simulink model "Copy_of_control_main"  (R2026a)
settings: Solver=VariableStepAuto  StopTime=inf  FixedStep=0.01
values from neighbouring files (symbols this model uses):
  coefficients = [20.111978783 20.2762923351 20.4770477048]    [sensor_calibration.mat]
undefined symbols (not defined in the file or in its folder): az, Q
libraries: instrumentseriallib x3
settings Model: Creator=user  LastModifiedBy=user

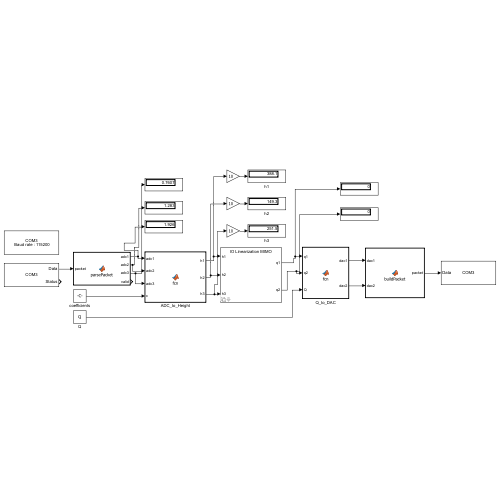
[thumbnail: Simulink's stored preview of the top-level diagram]
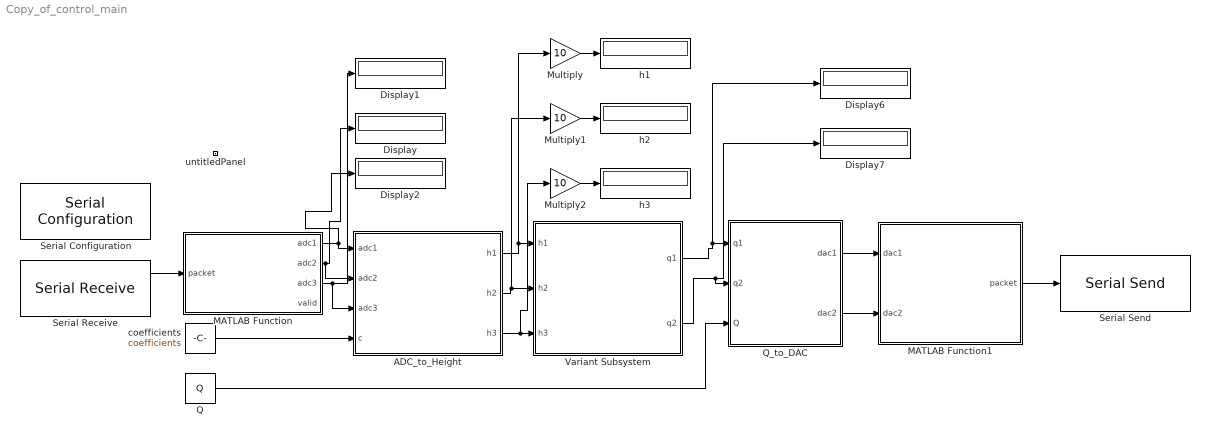
== system Copy_of_control_main ==
  ADC_to_Height : MATLAB Function  TreatAsAtomicUnit=on
  Display{,1..2,6..7} (5 alike) : Display
  MATLAB Function : MATLAB Function  TreatAsAtomicUnit=on
  MATLAB Function1 : MATLAB Function  TreatAsAtomicUnit=on
  Multiply : Gain  Gain=10
  Multiply1 : Gain  Gain=10
  Multiply2 : Gain  Gain=10
  Q : Constant  Value=Q
  Q_to_DAC : MATLAB Function  TreatAsAtomicUnit=on
  Serial Configuration : instrumentseriallib/Serial Configuration  Priority=-200000  PortSel=COM3  Port=COM3  ComPort=COM3  BaudRate=115200  DataBits=8  Parity=none  StopBits=1  ByteOrder=little-endian  FlowControl=none  Timeout=10  SimulateUsing=Interpreted execution  BlockInModel=on  aMode=1
  Serial Receive : instrumentseriallib/Serial Receive  Priority=1  PortSel=COM3  Port=COM3  ComPort=COM3  DataType=uint8  SaveDataType=uint8  ToggleHeader=on  Header=[0xAA 0x01]  ToggleDataSize=on  DataSize=[7]  ToggleTerminator=off  Terminator=<none>  CustomTerminator=[]  InputFormat=Column major  EnableBlockingMode=off  ActionDataUnavailable=Output last received value  ActionWhenDataUnavailable=Output last received value  CustomValue=0  SampleTime=0.01  SimulateUsing=Interpreted execution  BlockInModel=on  aMode=1  LibraryInUse=instrumentlib
  Serial Send : instrumentseriallib/Serial Send  Priority=1  PortSel=COM3  Port=COM3  ComPort=COM3  Header=[]  Terminator=<none>  CustomTerminator=[]  EnableBlockingMode=off  SimulateUsing=Interpreted execution  BlockInModel=on  aMode=1
  Variant Subsystem : Subsystem  Variant=on  mask{ctrl_mode=IO Linearization MIMO, r1=35, r2=25, r3=25, Kp_PI=10, Ki_PI=1, Kp1_PI=10, Ki1_PI=1, Kp2_PI=9, Ki2_PI=0.09, Kp_IO=0.5, Kp1_IO=1, Kp3_IO=15, Kp1_LIO=0, Kp3_LIO=0, Kd3_LIO=0, K_BS=1, Kz_BS=1, K1_BS=1, K3_BS=1, Kz_LBS=0, K1_LBS=0, K3_LBS=0, S1=10, S2=1, S3=10, R1_MPC=0.005, R2_MPC=0.005, H=40, S1_LMPC=10, S2_LMPC=1, S3_LMPC=10, R1_LMPC=0.005, R2_LMPC=0.005, H_LMPC=40}
      mask prompts: r1 "Tank1"; r2 "Tank2"; r3 "Tank3"; Kp_PI "Kp"; Ki_PI "Ki"; Kp1_PI "Kp1"; Ki1_PI "Ki1"; Kp2_PI "Kp2"; Ki2_PI "Ki2"; Kp_IO "Kp"; Kp1_IO "Kp1"; Kp3_IO "Kp3"; Kp1_LIO "Kp1"; Kp3_LIO "Kp3"; Kd3_LIO "Kd3"; K_BS "K"; Kz_BS "Kz"; K1_BS "K1"; K3_BS "K3"; Kz_LBS "Kz"; K1_LBS "K1"; K3_LBS "K3"; R1_MPC "R1"; R2_MPC "R2"; S1_LMPC "S1"; S2_LMPC "S2"; S3_LMPC "S3"; R1_LMPC "R1"; R2_LMPC "R2"; H_LMPC "H"
      mask DialogControl ParameterGroupVar Prompt: Controller
      mask DialogControl Container4 Prompt: Reference Levels
      mask DialogControl Container5 Prompt: PI SISO Parameters
      mask DialogControl Container6 Prompt: PI MIMO Parameters
      mask DialogControl Container7 Prompt: IO Linearization SISO
      mask DialogControl Container8 Prompt: IO Linearization MIMO
      mask DialogControl Container14 Prompt: Learning based IO Linearization MIMO
      mask DialogControl Container9 Prompt: Backstepping SISO
      mask DialogControl Container10 Prompt: Backstepping MIMO
      mask DialogControl Container13 Prompt: Learning based Backstepping MIMO
      mask DialogControl Container11 Prompt: MPC
      mask DialogControl Container12 Prompt: Learning based MPC
      mask DialogControl Container15 Prompt: RL
  coefficients : Constant  Value=coefficients
  h1 : Display
  h2 : Display
  h3 : Display
  untitledPanel : Subsystem  Tag=HiddenForWebPanel  IsWebBlockPanel=on
  wires:
  MATLAB Function1/1(packet) -> Serial Send/1
  Serial Receive/1 -> MATLAB Function/1(packet)
  MATLAB Function/2(adc2) -> ADC_to_Height/2(adc2), Display/1
  MATLAB Function/3(adc3) -> ADC_to_Height/3(adc3), Display1/1
  coefficients/1 -> ADC_to_Height/4(c)
  Q_to_DAC/1(dac1) -> MATLAB Function1/1(dac1)
  Q_to_DAC/2(dac2) -> MATLAB Function1/2(dac2)
  Q/1 -> Q_to_DAC/3(Q)
  ADC_to_Height/2(h2) -> Multiply1/1, Variant Subsystem/2(h2)
  ADC_to_Height/3(h3) -> Multiply2/1, Variant Subsystem/3(h3)
  Variant Subsystem/1(q1) -> Display6/1, Q_to_DAC/1(q1)
  Variant Subsystem/2(q2) -> Display7/1, Q_to_DAC/2(q2)
  MATLAB Function/1(adc1) -> ADC_to_Height/1(adc1), Display2/1
  Multiply/1 -> h1/1
  ADC_to_Height/1(h1) -> Multiply/1, Variant Subsystem/1(h1)
  Multiply1/1 -> h2/1
  Multiply2/1 -> h3/1

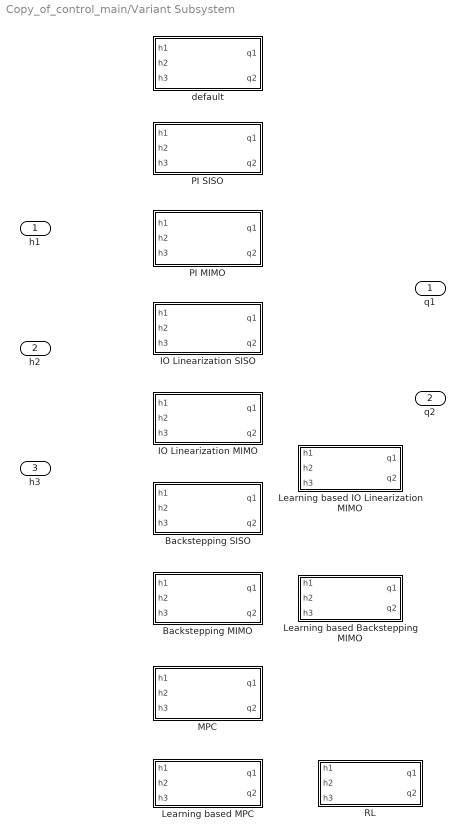
== system Copy_of_control_main/Variant Subsystem ==
  h1 : Inport
  h2 : Inport  Port=2
  h3 : Inport  Port=3
  Backstepping MIMO : Subsystem  VariantControl=ctrl_mode == 7
  Backstepping SISO : Subsystem  VariantControl=ctrl_mode == 6
  IO Linearization MIMO : Subsystem  VariantControl=ctrl_mode == 4
  IO Linearization SISO : Subsystem  VariantControl=ctrl_mode == 3
  Learning based Backstepping MIMO : Subsystem  VariantControl=ctrl_mode == 8
  Learning based IO Linearization MIMO : Subsystem  VariantControl=ctrl_mode == 5
  Learning based MPC : Subsystem  VariantControl=ctrl_mode == 10
  MPC : Subsystem  VariantControl=ctrl_mode == 9
  PI MIMO : Subsystem  VariantControl=ctrl_mode == 2
  PI SISO : Subsystem  VariantControl=ctrl_mode == 1
  RL : Subsystem  VariantControl=ctrl_mode == 11
  default : Subsystem  VariantControl=ctrl_mode == 0
  q1 : Outport
  q2 : Outport  Port=2

== system Copy_of_control_main/untitledPanel ==
  Dashboard Scope : DashboardScope  Tag=HiddenForWebPanel  PanelInfo="{\"height\":404,\"left\":393,\"panelId\":\"panelId-8aad0df7-f305-4620-9adc-6ae666dad641\",\"top\":27,\"type\":\"panelChild\",\"version\":\"2019b\",\"width\":464,\"zIndex\":1500004}"  Ymin=50  Ymax=550  FontColor=[0.0, 0.0, 0.0]
  Radio Button : RadioButtonGroup  Tag=HiddenForWebPanel  PanelInfo="{\"height\":384,\"left\":33,\"panelId\":\"panelId-8aad0df7-f305-4620-9adc-6ae666dad641\",\"top\":42,\"type\":\"panelChild\",\"version\":\"2019b\",\"width\":318,\"zIndex\":1500002}"  ButtonGroupName=Control Mode
  panelInfo : PanelWebBlock  Tag=HiddenForWebPanel  PanelInfo="{\"compacted\":true,\"height\":468,\"isActiveTab\":true,\"left\":782,\"name\":\"Panel\",\"panelId\":\"panelId-8aad0df7-f305-4620-9adc-6ae666dad641\",\"tabIndex\":0,\"tabbedSetId\":\"tabbedSet3175960063\",\"top\":92,\"type\":\"panel\",\"version\":\"2019b\",\"visible\":true,\"width\":881,\"zIndex\":1500002}"  PanelSnapshot=<binary blob, 100836 chars, not shown>

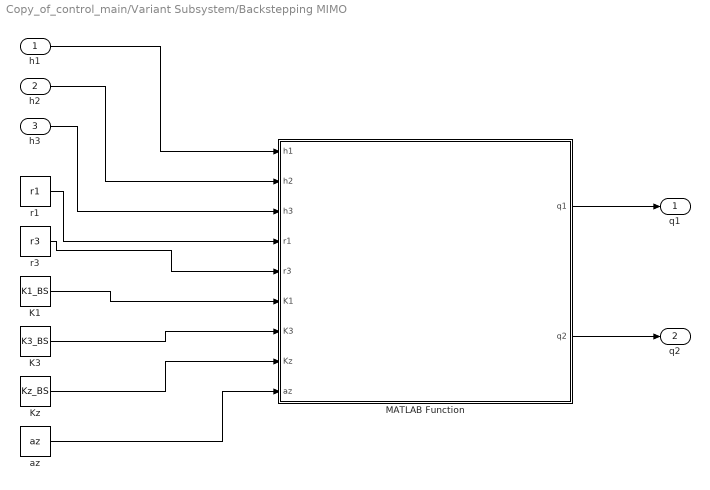
== system Copy_of_control_main/Variant Subsystem/Backstepping MIMO ==
  h1 : Inport
  h2 : Inport  Port=2
  h3 : Inport  Port=3
  K1 : Constant  Value=K1_BS
  K3 : Constant  Value=K3_BS
  Kz : Constant  Value=Kz_BS
  MATLAB Function : MATLAB Function  TreatAsAtomicUnit=on
  az : Constant  Value=az
  r1 : Constant  Value=r1
  r3 : Constant  Value=r3
  q1 : Outport
  q2 : Outport  Port=2
  wires:
  MATLAB Function/1(q1) -> q1/1
  MATLAB Function/2(q2) -> q2/1
  h1/1 -> MATLAB Function/1(h1)
  h2/1 -> MATLAB Function/2(h2)
  h3/1 -> MATLAB Function/3(h3)
  r1/1 -> MATLAB Function/4(r1)
  r3/1 -> MATLAB Function/5(r3)
  K1/1 -> MATLAB Function/6(K1)
  K3/1 -> MATLAB Function/7(K3)
  Kz/1 -> MATLAB Function/8(Kz)
  az/1 -> MATLAB Function/9(az)

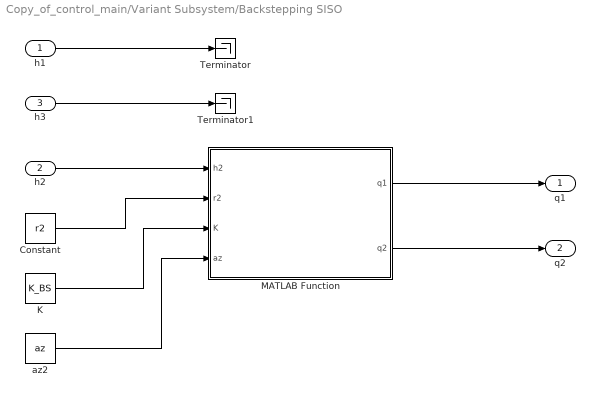
== system Copy_of_control_main/Variant Subsystem/Backstepping SISO ==
  h1 : Inport
  h2 : Inport  Port=2
  h3 : Inport  Port=3
  Constant : Constant  Value=r2
  K : Constant  Value=K_BS
  MATLAB Function : MATLAB Function  TreatAsAtomicUnit=on
  Terminator : Terminator
  Terminator1 : Terminator
  az2 : Constant  Value=az
  q1 : Outport
  q2 : Outport  Port=2
  wires:
  Constant/1 -> MATLAB Function/2(r2)
  az2/1 -> MATLAB Function/4(az)
  MATLAB Function/1(q1) -> q1/1
  MATLAB Function/2(q2) -> q2/1
  K/1 -> MATLAB Function/3(K)
  h3/1 -> Terminator1/1
  h2/1 -> MATLAB Function/1(h2)
  h1/1 -> Terminator/1

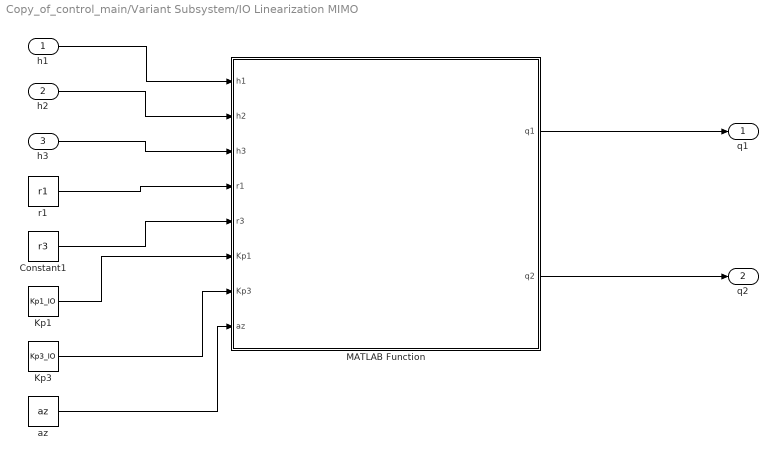
== system Copy_of_control_main/Variant Subsystem/IO Linearization MIMO ==
  h1 : Inport
  h2 : Inport  Port=2
  h3 : Inport  Port=3
  Constant1 : Constant  Value=r3
  Kp1 : Constant  Value=Kp1_IO
  Kp3 : Constant  Value=Kp3_IO
  MATLAB Function : MATLAB Function  TreatAsAtomicUnit=on
  az : Constant  Value=az
  r1 : Constant  Value=r1
  q1 : Outport
  q2 : Outport  Port=2
  wires:
  h2/1 -> MATLAB Function/2(h2)
  MATLAB Function/2(q2) -> q2/1
  MATLAB Function/1(q1) -> q1/1
  h1/1 -> MATLAB Function/1(h1)
  h3/1 -> MATLAB Function/3(h3)
  r1/1 -> MATLAB Function/4(r1)
  Constant1/1 -> MATLAB Function/5(r3)
  Kp1/1 -> MATLAB Function/6(Kp1)
  Kp3/1 -> MATLAB Function/7(Kp3)
  az/1 -> MATLAB Function/8(az)

== system Copy_of_control_main/Variant Subsystem/IO Linearization SISO ==
  h1 : Inport
  h2 : Inport  Port=2
  h3 : Inport  Port=3
  Kp : Constant  Value=Kp_IO
  MATLAB Function : MATLAB Function  TreatAsAtomicUnit=on
  Terminator : Terminator
  Terminator1 : Terminator
  az : Constant  Value=az
  r2 : Constant  Value=r2
  q1 : Outport
  q2 : Outport  Port=2
  wires:
  h2/1 -> MATLAB Function/1(h2)
  r2/1 -> MATLAB Function/2(r2)
  Kp/1 -> MATLAB Function/3(Kp)
  MATLAB Function/1(q1) -> q1/1
  MATLAB Function/2(q2) -> q2/1
  az/1 -> MATLAB Function/4(az)
  h1/1 -> Terminator/1
  h3/1 -> Terminator1/1

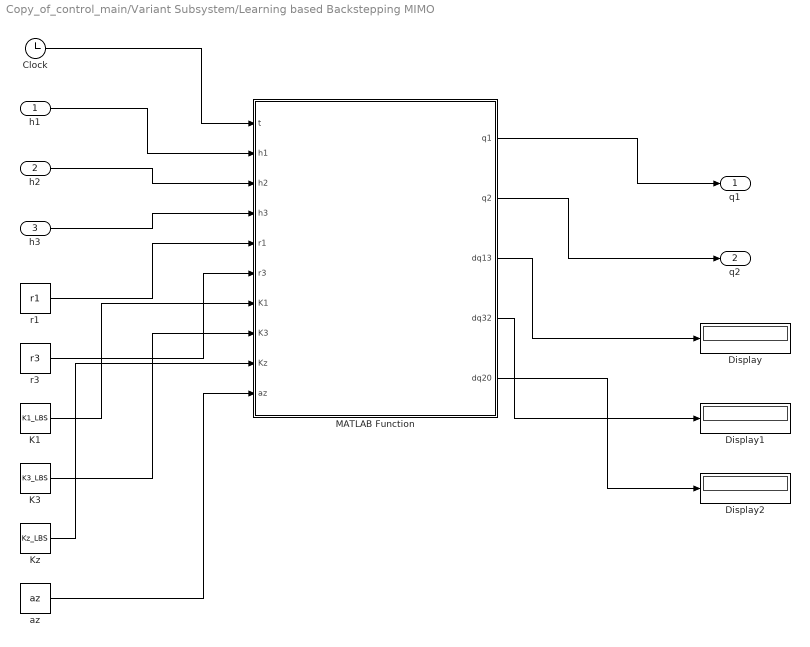
== system Copy_of_control_main/Variant Subsystem/Learning based Backstepping MIMO ==
  h1 : Inport
  h2 : Inport  Port=2
  h3 : Inport  Port=3
  Clock : Clock
  Display : Display
  Display1 : Display
  Display2 : Display
  K1 : Constant  Value=K1_LBS
  K3 : Constant  Value=K3_LBS
  Kz : Constant  Value=Kz_LBS
  MATLAB Function : MATLAB Function  TreatAsAtomicUnit=on
  az : Constant  Value=az
  r1 : Constant  Value=r1
  r3 : Constant  Value=r3
  q1 : Outport
  q2 : Outport  Port=2
  wires:
  MATLAB Function/1(q1) -> q1/1
  MATLAB Function/2(q2) -> q2/1
  h1/1 -> MATLAB Function/2(h1)
  h2/1 -> MATLAB Function/3(h2)
  h3/1 -> MATLAB Function/4(h3)
  r1/1 -> MATLAB Function/5(r1)
  r3/1 -> MATLAB Function/6(r3)
  K1/1 -> MATLAB Function/7(K1)
  K3/1 -> MATLAB Function/8(K3)
  Kz/1 -> MATLAB Function/9(Kz)
  az/1 -> MATLAB Function/10(az)
  MATLAB Function/3(dq13) -> Display/1
  MATLAB Function/4(dq32) -> Display1/1
  MATLAB Function/5(dq20) -> Display2/1
  Clock/1 -> MATLAB Function/1(t)

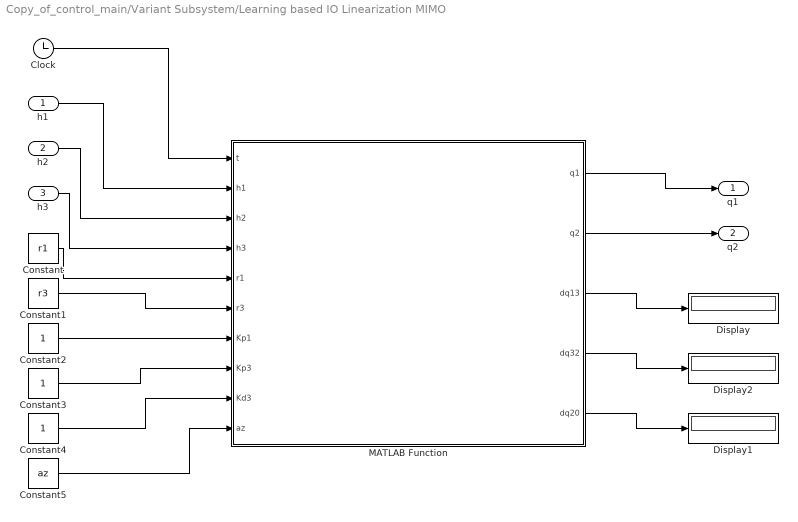
== system Copy_of_control_main/Variant Subsystem/Learning based IO Linearization MIMO ==
  h1 : Inport
  h2 : Inport  Port=2
  h3 : Inport  Port=3
  Clock : Clock
  Constant : Constant  Value=r1
  Constant1 : Constant  Value=r3
  Constant2 : Constant
  Constant3 : Constant
  Constant4 : Constant
  Constant5 : Constant  Value=az
  Display : Display
  Display1 : Display
  Display2 : Display
  MATLAB Function : MATLAB Function  TreatAsAtomicUnit=on
  q1 : Outport
  q2 : Outport  Port=2
  wires:
  h1/1 -> MATLAB Function/2(h1)
  h2/1 -> MATLAB Function/3(h2)
  h3/1 -> MATLAB Function/4(h3)
  Constant/1 -> MATLAB Function/5(r1)
  Constant1/1 -> MATLAB Function/6(r3)
  Constant2/1 -> MATLAB Function/7(Kp1)
  Constant3/1 -> MATLAB Function/8(Kp3)
  Constant4/1 -> MATLAB Function/9(Kd3)
  Constant5/1 -> MATLAB Function/10(az)
  MATLAB Function/1(q1) -> q1/1
  MATLAB Function/2(q2) -> q2/1
  Clock/1 -> MATLAB Function/1(t)
  MATLAB Function/3(dq13) -> Display/1
  MATLAB Function/4(dq32) -> Display2/1
  MATLAB Function/5(dq20) -> Display1/1

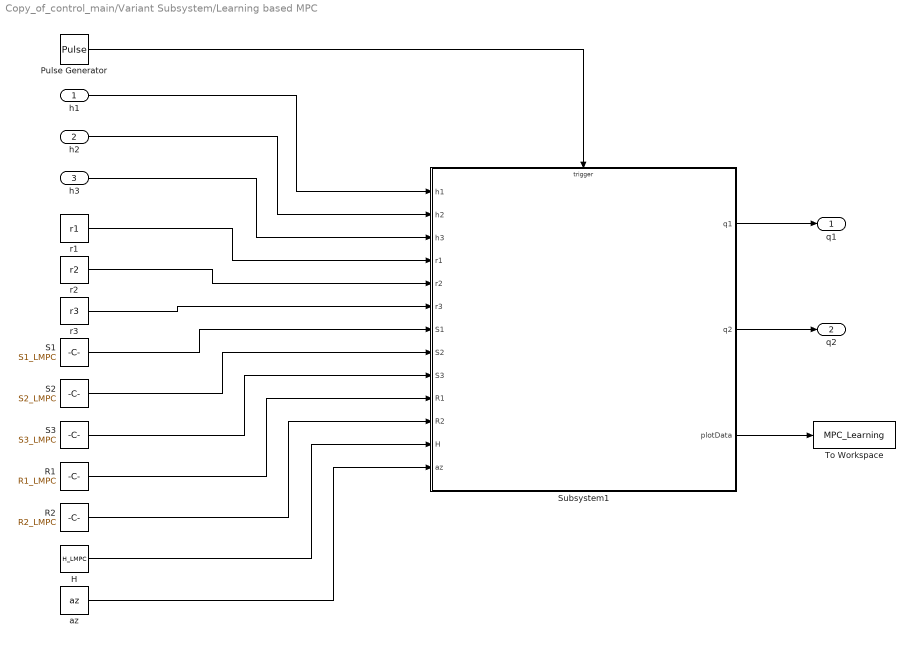
== system Copy_of_control_main/Variant Subsystem/Learning based MPC ==
  h1 : Inport
  h2 : Inport  Port=2
  h3 : Inport  Port=3
  H : Constant  Value=H_LMPC
  Pulse Generator : DiscretePulseGenerator  Period=5  SampleTime=0.01
  R1 : Constant  Value=R1_LMPC
  R2 : Constant  Value=R2_LMPC
  S1 : Constant  Value=S1_LMPC
  S2 : Constant  Value=S2_LMPC
  S3 : Constant  Value=S3_LMPC
  Subsystem1 : Subsystem
  To Workspace : ToWorkspace  VariableName=MPC_Learning  SaveFormat=Timeseries  SampleTime=-1
  az : Constant  Value=az
  r1 : Constant  Value=r1
  r2 : Constant  Value=r2
  r3 : Constant  Value=r3
  q1 : Outport
  q2 : Outport  Port=2
  wires:
  h1/1 -> Subsystem1/1(h1)
  h2/1 -> Subsystem1/2(h2)
  h3/1 -> Subsystem1/3(h3)
  r1/1 -> Subsystem1/4(r1)
  r2/1 -> Subsystem1/5(r2)
  r3/1 -> Subsystem1/6(r3)
  S1/1 -> Subsystem1/7(S1)
  S2/1 -> Subsystem1/8(S2)
  S3/1 -> Subsystem1/9(S3)
  R1/1 -> Subsystem1/10(R1)
  R2/1 -> Subsystem1/11(R2)
  H/1 -> Subsystem1/12(H)
  az/1 -> Subsystem1/13(az)
  Subsystem1/1(q1) -> q1/1
  Subsystem1/2(q2) -> q2/1
  Subsystem1/3(plotData) -> To Workspace/1
  Pulse Generator/1 -> Subsystem1/Trigger

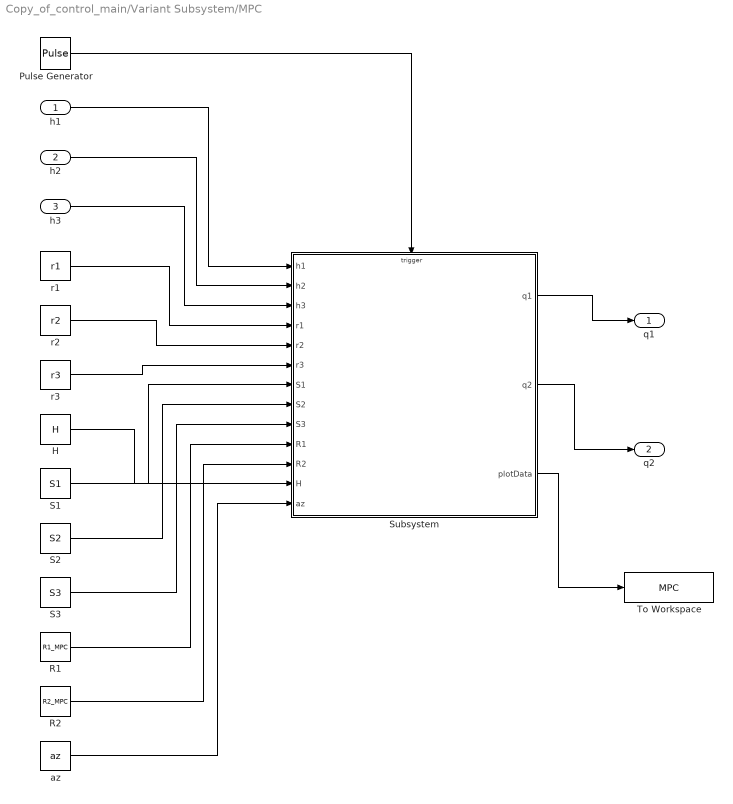
== system Copy_of_control_main/Variant Subsystem/MPC ==
  h1 : Inport
  h2 : Inport  Port=2
  h3 : Inport  Port=3
  H : Constant  Value=H
  Pulse Generator : DiscretePulseGenerator  Period=5  SampleTime=0.01
  R1 : Constant  Value=R1_MPC
  R2 : Constant  Value=R2_MPC
  S1 : Constant  Value=S1
  S2 : Constant  Value=S2
  S3 : Constant  Value=S3
  Subsystem : Subsystem
  To Workspace : ToWorkspace  VariableName=MPC  SaveFormat=Timeseries  SampleTime=-1
  az : Constant  Value=az
  r1 : Constant  Value=r1
  r2 : Constant  Value=r2
  r3 : Constant  Value=r3
  q1 : Outport
  q2 : Outport  Port=2
  wires:
  h1/1 -> Subsystem/1(h1)
  h2/1 -> Subsystem/2(h2)
  h3/1 -> Subsystem/3(h3)
  r1/1 -> Subsystem/4(r1)
  r2/1 -> Subsystem/5(r2)
  r3/1 -> Subsystem/6(r3)
  S1/1 -> Subsystem/7(S1)
  S2/1 -> Subsystem/8(S2)
  S3/1 -> Subsystem/9(S3)
  R1/1 -> Subsystem/10(R1)
  R2/1 -> Subsystem/11(R2)
  H/1 -> Subsystem/12(H)
  az/1 -> Subsystem/13(az)
  Subsystem/1(q1) -> q1/1
  Subsystem/2(q2) -> q2/1
  Subsystem/3(plotData) -> To Workspace/1
  Pulse Generator/1 -> Subsystem/Trigger

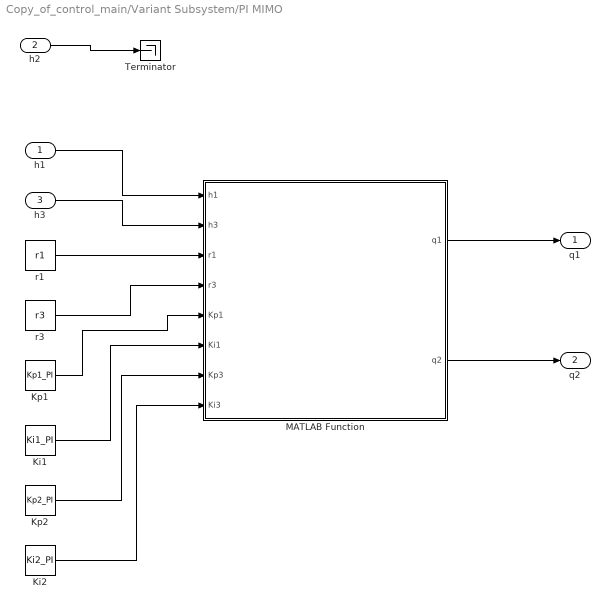
== system Copy_of_control_main/Variant Subsystem/PI MIMO ==
  h1 : Inport
  h2 : Inport  Port=2
  h3 : Inport  Port=3
  Ki1 : Constant  Value=Ki1_PI
  Ki2 : Constant  Value=Ki2_PI
  Kp1 : Constant  Value=Kp1_PI
  Kp2 : Constant  Value=Kp2_PI
  MATLAB Function : MATLAB Function  TreatAsAtomicUnit=on
  Terminator : Terminator
  r1 : Constant  Value=r1
  r3 : Constant  Value=r3
  q1 : Outport
  q2 : Outport  Port=2
  wires:
  MATLAB Function/2(q2) -> q2/1
  MATLAB Function/1(q1) -> q1/1
  h1/1 -> MATLAB Function/1(h1)
  h3/1 -> MATLAB Function/2(h3)
  r1/1 -> MATLAB Function/3(r1)
  r3/1 -> MATLAB Function/4(r3)
  Kp1/1 -> MATLAB Function/5(Kp1)
  Ki1/1 -> MATLAB Function/6(Ki1)
  Kp2/1 -> MATLAB Function/7(Kp3)
  Ki2/1 -> MATLAB Function/8(Ki3)
  h2/1 -> Terminator/1

== system Copy_of_control_main/Variant Subsystem/PI SISO ==
  h1 : Inport
  h2 : Inport  Port=2
  h3 : Inport  Port=3
  Constant : Constant  Value=r2
  Ki : Constant  Value=Ki_PI
  Kp : Constant  Value=Kp_PI
  MATLAB Function : MATLAB Function  TreatAsAtomicUnit=on
  Terminator : Terminator
  Terminator1 : Terminator
  q1 : Outport
  q2 : Outport  Port=2
  wires:
  MATLAB Function/2(q2) -> q2/1
  MATLAB Function/1(q1) -> q1/1
  h2/1 -> MATLAB Function/1(h2)
  Constant/1 -> MATLAB Function/2(r2)
  Kp/1 -> MATLAB Function/3(Kp)
  Ki/1 -> MATLAB Function/4(Ki)
  h1/1 -> Terminator/1
  h3/1 -> Terminator1/1

== system Copy_of_control_main/Variant Subsystem/RL ==
  h1 : Inport
  h2 : Inport  Port=2
  h3 : Inport  Port=3
  " RL" : MATLAB Function  TreatAsAtomicUnit=on
  r1 : Constant  Value=r1
  r2 : Constant  Value=r2
  r3 : Constant  Value=r3
  q1 : Outport
  q2 : Outport  Port=2
  wires:
  r3/1 -> " RL"/6(r3)
  r2/1 -> " RL"/5(r2)
  r1/1 -> " RL"/4(r1)
  h3/1 -> " RL"/3(h3)
  h2/1 -> " RL"/2(h2)
  h1/1 -> " RL"/1(h1)
  " RL"/2(q2) -> q2/1
  " RL"/1(q1) -> q1/1

== system Copy_of_control_main/Variant Subsystem/default ==
  h1 : Inport
  h2 : Inport  Port=2
  h3 : Inport  Port=3
  Constant : Constant  Value=0
  Constant1 : Constant  Value=0
  Terminator : Terminator
  Terminator1 : Terminator
  Terminator2 : Terminator
  q1 : Outport
  q2 : Outport  Port=2
  wires:
  Constant/1 -> q1/1
  Constant1/1 -> q2/1
  h1/1 -> Terminator/1
  h2/1 -> Terminator1/1
  h3/1 -> Terminator2/1

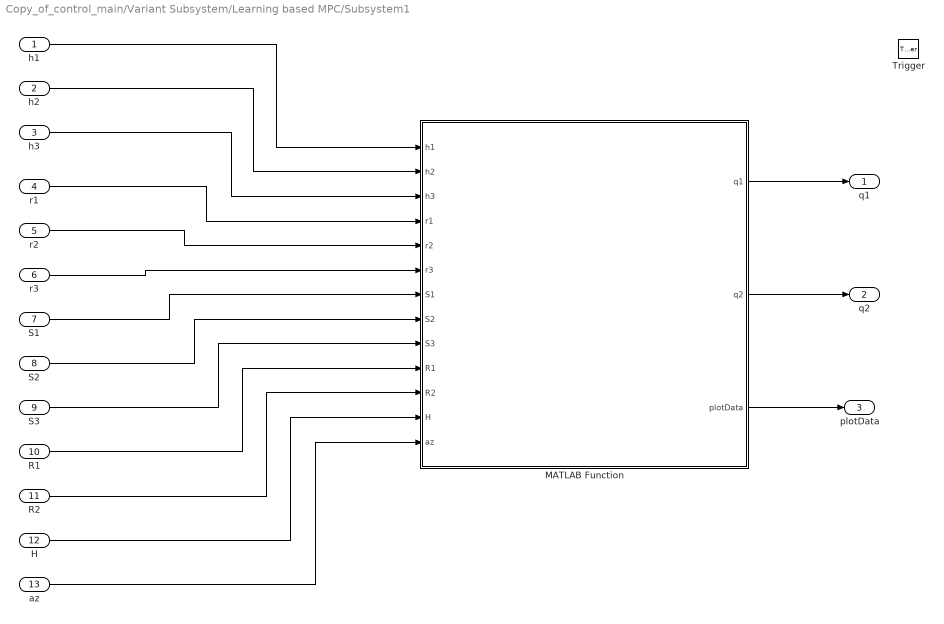
== system Copy_of_control_main/Variant Subsystem/Learning based MPC/Subsystem1 ==
  h1 : Inport
  h2 : Inport  Port=2
  h3 : Inport  Port=3
  r1 : Inport  Port=4
  r2 : Inport  Port=5
  r3 : Inport  Port=6
  S1 : Inport  Port=7
  S2 : Inport  Port=8
  S3 : Inport  Port=9
  R1 : Inport  Port=10
  R2 : Inport  Port=11
  H : Inport  Port=12
  az : Inport  Port=13
  Trigger : TriggerPort  VariantControl=(inherit)  PortDimensions=1
  MATLAB Function : MATLAB Function  TreatAsAtomicUnit=on
  q1 : Outport
  q2 : Outport  Port=2
  plotData : Outport  Port=3
  wires:
  MATLAB Function/1(q1) -> q1/1
  MATLAB Function/2(q2) -> q2/1
  MATLAB Function/3(plotData) -> plotData/1
  h1/1 -> MATLAB Function/1(h1)
  S1/1 -> MATLAB Function/7(S1)
  r1/1 -> MATLAB Function/4(r1)
  S3/1 -> MATLAB Function/9(S3)
  H/1 -> MATLAB Function/12(H)
  az/1 -> MATLAB Function/13(az)
  S2/1 -> MATLAB Function/8(S2)
  r2/1 -> MATLAB Function/5(r2)
  R2/1 -> MATLAB Function/11(R2)
  r3/1 -> MATLAB Function/6(r3)
  h3/1 -> MATLAB Function/3(h3)
  R1/1 -> MATLAB Function/10(R1)
  h2/1 -> MATLAB Function/2(h2)

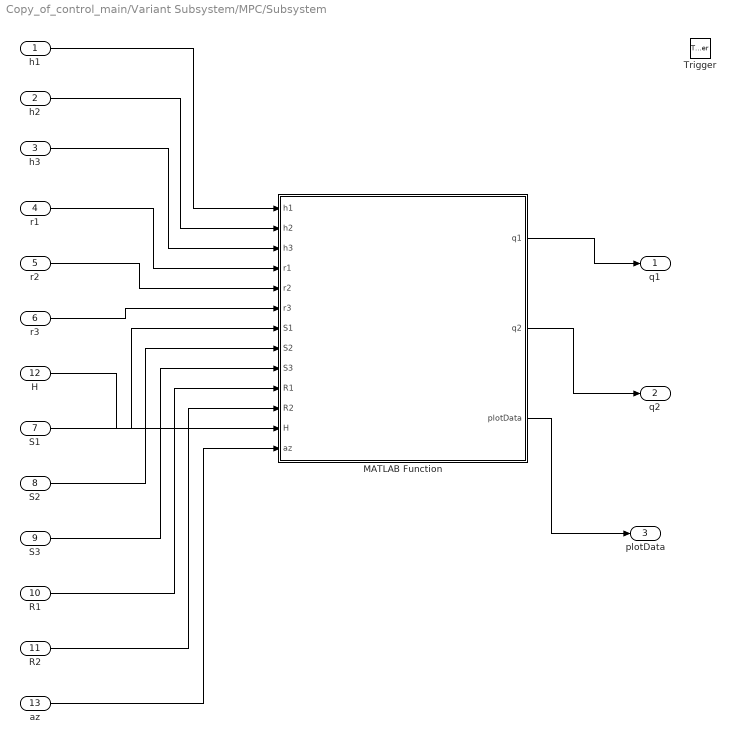
== system Copy_of_control_main/Variant Subsystem/MPC/Subsystem ==
  h1 : Inport
  h2 : Inport  Port=2
  h3 : Inport  Port=3
  r1 : Inport  Port=4
  r2 : Inport  Port=5
  r3 : Inport  Port=6
  S1 : Inport  Port=7
  S2 : Inport  Port=8
  S3 : Inport  Port=9
  R1 : Inport  Port=10
  R2 : Inport  Port=11
  H : Inport  Port=12
  az : Inport  Port=13
  Trigger : TriggerPort  VariantControl=(inherit)  PortDimensions=1
  MATLAB Function : MATLAB Function  TreatAsAtomicUnit=on
  q1 : Outport
  q2 : Outport  Port=2
  plotData : Outport  Port=3
  wires:
  R1/1 -> MATLAB Function/10(R1)
  h3/1 -> MATLAB Function/3(h3)
  MATLAB Function/1(q1) -> q1/1
  MATLAB Function/3(plotData) -> plotData/1
  r3/1 -> MATLAB Function/6(r3)
  r2/1 -> MATLAB Function/5(r2)
  MATLAB Function/2(q2) -> q2/1
  R2/1 -> MATLAB Function/11(R2)
  r1/1 -> MATLAB Function/4(r1)
  S1/1 -> MATLAB Function/7(S1)
  S2/1 -> MATLAB Function/8(S2)
  H/1 -> MATLAB Function/12(H)
  S3/1 -> MATLAB Function/9(S3)
  h2/1 -> MATLAB Function/2(h2)
  az/1 -> MATLAB Function/13(az)
  h1/1 -> MATLAB Function/1(h1)

== matlab function Copy_of_control_main/Variant Subsystem/IO Linearization MIMO/MATLAB Function ==
  data: h1 input; q1 output; h2 input; h3 input; r1 input; r3 input; Kp1 input; Kp3 input; az input; q2 output
function [q1,q2] = IO_MIMO(h1,h2,h3,r1,r3,Kp1,Kp3,az)

A = 154.0;
Sn = 0.5;
g = 981.0;

az1 = az(1);
az2 = az(2);
az3 = az(3);

c1 = az1 * Sn;
c2 = az2 * Sn;
c3 = az3 * Sn;

q13 = c1 * sign(h1-h3) * sqrt(2*g*abs(h1-h3));
q32 = c3 * sign(h3-h2) * sqrt(2*g*abs(h3-h2));
q20 = c2 * sqrt(2*g*max(h2,0));

e1 = r1 - h1;
v1 = Kp1 * e1;

q1 = A*v1 + q13;
q1 = min(max(q1,0),85);

Kd3 = sqrt(2*Kp3);

e3 = r3 - h3;
dh3 = (q13 - q32)/A;

v2 = Kp3*e3 - Kd3*dh3;

den13 = sqrt(abs(h1-h3));
den32 = sqrt(abs(h3-h2));

EPS_DEN = 1e-3;
den13_safe = max(den13,EPS_DEN);

term1 = -(c1*den32)/(c3*den13_safe) ...
        * (q1 - 2*q13 + q32);

term2 = q13 - 2*q32 + q20;

term3 = sqrt(2*g*abs(h3-h2))/(c3*g) ...
        * A^2 * v2;

q2 = term1 + term2 + term3;

q2 = min(max(q2,0),85);

end

== matlab function Copy_of_control_main/Variant Subsystem/Backstepping SISO/MATLAB Function ==
  data: h2 input; q1 output; r2 input; K input; az input; q2 output
function [q1,q2] = Backstepping_SISO(h2,r2,K,az)
% backstepping误差指数减小  de/dt=-Ke​

A  = 154.0;
Sn = 0.5;
g  = 981.0;
Ofc2 = az(2);

q20 = Ofc2 * Sn * sqrt(2*g*max(h2,0));

q1 = 0;
q2 = q20 + A*K*(r2 - h2);

q2 = min(max(q2,0),85);

end

== matlab function Copy_of_control_main/Variant Subsystem/Backstepping MIMO/MATLAB Function ==
  data: h1 input; q1 output; h2 input; h3 input; r1 input; r3 input; K1 input; K3 input; Kz input; az input; q2 output
function [q1,q2] = Backstepping_MIMO(h1,h2,h3,r1,r3,K1,K3,Kz,az)
% Backstepping MIMO for Tank1 and Tank3
% K1       : Tank1 error gain
% K3       : Tank3 virtual control gain
% Kz       : q32 tracking gain


A  = 154.0;
Sn = 0.5;
g  = 981.0;
TWOG = 2*g;
epsv = 1e-6;

az1 = az(1);
az2 = az(2);
az3 = az(3);

q13 = az1 * Sn * sqrt(TWOG * max(h1-h3, 0));
q32 = az3 * Sn * sqrt(TWOG * max(h3-h2, 0));
q20 = az2 * Sn * sqrt(TWOG * max(h2,    0));

% if r1 == 0 && r3 == 0
%     q1 = 0;
%     q2 = 0;
%     return;
% else
% end
% Step 1: control h1
% e1 = h1 - r1, desired e1_dot = -K1*e1
% q1 = q13 - A*K1*e1

e1 = h1 - r1;

q1 = q13 - A*K1*e1;
q1 = min(max(q1,0),85);

% Step 2: virtual control for h3
% e3 = h3 - r3
% desired e3_dot = -K3*e3
% q32_des = q13 + A*K3*e3
e3 = h3 - r3;

q32_des = q13 + A*K3*e3;

% virtual tracking error
z = q32 - q32_des;

% Compute derivative of q32_des
% q32_des_dot = q13_dot + A*K3*e3_dot
% e3_dot = h3_dot = (q13-q32)/A
% q13_dot = k13*(h1_dot-h3_dot)
dh13 = max(h1-h3, epsv);
dh32 = max(h3-h2, epsv);

k13 = (az1 * Sn * TWOG) / (2 * sqrt(TWOG * dh13));
k32 = (az3 * Sn * TWOG) / (2 * sqrt(TWOG * dh32));

h1_dot = (q1 - q13) / A;
h3_dot = (q13 - q32) / A;

q13_dot = k13 * (h1_dot - h3_dot);

q32_des_dot = q13_dot + A*K3*h3_dot;

% Step 3: real control q2
% z_dot = -Kz*z
%
% q2 = q13 - 2*q32 + q20
%      - (A/k32)*q32_des_dot
%      + (A/k32)*Kz*z
q2 = q13 - 2*q32 + q20 ...
     - (A/k32)*q32_des_dot ...
     + (A/k32)*Kz*z;

q2 = min(max(q2,0),85);

end

== matlab function Copy_of_control_main/Variant Subsystem/MPC/Subsystem/MATLAB Function ==
  data: h1 input; q1 output; h2 input; h3 input; r1 input; r2 input; r3 input; S1 input; S2 input; S3 input; R1 input; R2 input; H input; q2 output; az input size=[1 3]; plotData output
function [q1,q2,plotData] = MPC( ...
    h1,h2,h3, ...
    r1,r2,r3, ...
    S1,S2,S3, ...
    R1,R2,H,az)

A    = 154.0;
Sn   = 0.5;
g    = 981.0;
Ts   = 0.05;
Qmax = 85.0;

nx   = 3;
nu   = 2;
ny   = 3;
Hmax = 40;

Niter = 200;

persistent uPrevious

if isempty(uPrevious)
    uPrevious = zeros(2,1);
end


H = round(H);

if H < 1
    H = 1;
elseif H > Hmax
    H = Hmax;
end

az1 = az(1);
az2 = az(2);
az3 = az(3);

C1 = az1*Sn;
C2 = az3*Sn;
C3 = az2*Sn;


x = [h1;h2;h3];
r = [r1;r2;r3];


xbar = max(x,0.1);
ubar = zeros(2,1);

[Ad,Bd,dd] = linearModelAffine( ...
    xbar,ubar,Ts,A,C1,C2,C3,g);


Phi   = zeros(ny*H,nx);
Gamma = zeros(ny*H,nu*H);
Dbar  = zeros(ny*H,1);

Ai = eye(nx);
di = zeros(nx,1);

for i = 1:H

    Ai = Ai*Ad;
    di = Ad*di + dd;

    row1 = (i-1)*ny + 1;
    row2 = i*ny;

    Phi(row1:row2,:) = Ai;
    Dbar(row1:row2)  = di;

    for j = 1:i

        col1 = (j-1)*nu + 1;
        col2 = j*nu;

        Aij = eye(nx);

        for k = 1:(i-j)
            Aij = Aij*Ad;
        end

        Gamma(row1:row2,col1:col2) = Aij*Bd;
    end
end


S = diag([S1 S2 S3]);
R = diag([R1 R2]);

Sbar = zeros(ny*H,ny*H);
Rbar = zeros(nu*H,nu*H);

for i = 1:H

    sy1 = (i-1)*ny + 1;
    sy2 = i*ny;

    ru1 = (i-1)*nu + 1;
    ru2 = i*nu;

    Sbar(sy1:sy2,sy1:sy2) = S;
    Rbar(ru1:ru2,ru1:ru2) = R;
end

Rref = zeros(ny*H,1);

for i = 1:H

    row1 = (i-1)*ny + 1;
    row2 = i*ny;

    Rref(row1:row2) = r;
end

Xfree = Phi*x + Dbar;


Dmat = zeros(nu*H,nu*H);
UpreviousBar = zeros(nu*H,1);

for i = 1:H

    row1 = (i-1)*nu + 1;
    row2 = i*nu;

    Dmat(row1:row2,row1:row2) = eye(nu);

    if i == 1

        UpreviousBar(row1:row2) = uPrevious;

    else

        col1 = (i-2)*nu + 1;
        col2 = (i-1)*nu;

        Dmat(row1:row2,col1:col2) = -eye(nu);
    end
end

regularization = 1e-8;

G = Gamma'*Sbar*Gamma ...
    + Dmat'*Rbar*Dmat ...
    + regularization*eye(nu*H);

F = Gamma'*Sbar*(Xfree-Rref) ...
    - Dmat'*Rbar*UpreviousBar;

G = 0.5*(G+G');


U = zeros(nu*H,1);

maxRowSum = 0.0;

for i = 1:(nu*H)

    rowSum = 0.0;

    for j = 1:(nu*H)
        rowSum = rowSum + abs(G(i,j));
    end

    if rowSum > maxRowSum
        maxRowSum = rowSum;
    end
end

alpha = 1.0/max(maxRowSum,1e-9);

for iter = 1:Niter

    grad = G*U + F;

    Unew = U - alpha*grad;

    for k = 1:(nu*H)

        if Unew(k) < 0.0
            Unew(k) = 0.0;

        elseif Unew(k) > Qmax
            Unew(k) = Qmax;
        end
    end

    U = Unew;
end


q1 = U(1);
q2 = U(2);

uPrevious = [q1;q2];


plotData = zeros(9,1);

plotData(1) = h1;
plotData(2) = h2;
plotData(3) = h3;

plotData(4) = r1;
plotData(5) = r2;
plotData(6) = r3;

plotData(7) = q1;
plotData(8) = q2;
plotData(9) = alpha;

end


function [Ad,Bd,dd] = linearModelAffine( ...
    xbar,ubar,Ts,A,C1,C2,C3,g)

epsv = 1e-6;

h1 = max(xbar(1),0.0);
h2 = max(xbar(2),0.0);
h3 = max(xbar(3),0.0);

d13 = h1-h3;
d32 = h3-h2;

absD13 = max(abs(d13),epsv);
absD32 = max(abs(d32),epsv);
h2safe = max(h2,epsv);

k13 = C1*g/sqrt(2.0*g*absD13);
k32 = C2*g/sqrt(2.0*g*absD32);
k20 = C3*g/sqrt(2.0*g*h2safe);

Ac = zeros(3,3);

Ac(1,1) = -k13/A;
Ac(1,3) =  k13/A;

Ac(2,2) = (-k32-k20)/A;
Ac(2,3) =  k32/A;

Ac(3,1) =  k13/A;
Ac(3,2) =  k32/A;
Ac(3,3) = (-k13-k32)/A;

Bc = [1.0/A  0.0;
      0.0    1.0/A;
      0.0    0.0];

Ad = eye(3) + Ts*Ac;
Bd = Ts*Bc;

fbar = nonlinearDynamics( ...
    xbar,ubar,A,C1,C2,C3,g);

dd = xbar + Ts*fbar ...
    - Ad*xbar ...
    - Bd*ubar;

end


function xdot = nonlinearDynamics( ...
    x,u,A,C1,C2,C3,g)

h1 = max(x(1),0.0);
h2 = max(x(2),0.0);
h3 = max(x(3),0.0);

d13 = h1-h3;
d32 = h3-h2;

q13 = C1*sign(d13)*sqrt(2.0*g*abs(d13));
q32 = C2*sign(d32)*sqrt(2.0*g*abs(d32));
q20 = C3*sqrt(2.0*g*h2);

xdot = zeros(3,1);

xdot(1) = (u(1)-q13)/A;
xdot(2) = (u(2)+q32-q20)/A;
xdot(3) = (q13-q32)/A;

end

== matlab function Copy_of_control_main/Variant Subsystem/Learning based MPC/Subsystem1/MATLAB Function ==
  data: h1 input; q1 output; h2 input; h3 input; r1 input; r2 input; r3 input; S1 input; S2 input; S3 input; R1 input; R2 input; H input; az input; q2 output; plotData output
function [q1,q2,plotData] = MPC_Learning(h1,h2,h3,...
                                r1,r2,r3,...
                                S1,S2,S3,...
                                R1,R2,H,az)
%#codegen

A    = 154.0;
Sn   = 0.5;
g    = 981.0;
Ts   = 0.05;
Qmax = 85.0;

nx   = 3;
nu   = 2;
ny   = 3;
Hmax = 40;

learningrate         = 0.05;
residualLimit = 5.0;
Niter        = 200;

persistent residualHat xPredPrevious initialized uPrevious predictionErrorMean

if isempty(initialized)
    residualHat  = zeros(3,1);
    xPredPrevious = zeros(3,1);
    uPrevious     = zeros(2,1);
    predictionErrorMean = zeros(3,1);
    initialized  = false;
end

H = round(H);

if H < 1
    H = 1;
elseif H > Hmax
    H = Hmax;
end

az1 = az(1);
az2 = az(2);
az3 = az(3);

C1 = az1 * Sn;
C2 = az3 * Sn;
C3 = az2 * Sn;

x = [h1;h2;h3];
r = [r1;r2;r3];
predictionError = zeros(3,1);

% e(k) = x(k) - xPred(k|k-1)
% residualHat(k) = residualHat(k-1) + beta*e(k)

if initialized

    predictionError = x - xPredPrevious;

    tauError = 1.0;   
    alphaMA = Ts/(tauError + Ts);

    predictionErrorMean = ...
        (1.0-alphaMA)*predictionErrorMean ...
        + alphaMA*predictionError;

    residualHat = ...
        (1.0-learningrate)*residualHat ...
        + learningrate*predictionErrorMean;

    for i = 1:nx
        if residualHat(i) > residualLimit
            residualHat(i) = residualLimit;
        elseif residualHat(i) < -residualLimit
            residualHat(i) = -residualLimit;
        end
    end

else
    initialized = true;
end

xbar = max(x,0.1);
ubar = zeros(2,1);

[Ad,Bd,dd] = linearModelAffine(...
    xbar,ubar,Ts,A,C1,C2,C3,g);

% x(k+1) = Ad*x(k) + Bd*u(k) + dd + residualHat

dLearned = dd + residualHat;

% X = Phi*x + Gamma*U + Dbar

Phi   = zeros(ny*H,nx);
Gamma = zeros(ny*H,nu*H);
Dbar  = zeros(ny*H,1);

Ai = eye(nx);
di = zeros(nx,1);

for i = 1:H

    Ai = Ai*Ad;
    di = Ad*di + dLearned;

    row1 = (i-1)*ny + 1;
    row2 = i*ny;

    Phi(row1:row2,:) = Ai;
    Dbar(row1:row2) = di;

    for j=1:i

        col1 = (j-1)*nu + 1;
        col2 = j*nu;

        Aij = eye(nx);

        for k=1:(i-j)
            Aij = Aij*Ad;
        end

        Gamma(row1:row2,col1:col2)=Aij*Bd;

    end
end

S = diag([S1 S2 S3]);

R = diag([R1 R2]);

Sbar = zeros(ny*H,ny*H);
Rbar = zeros(nu*H,nu*H);

for i = 1:H

    sy1 = (i-1)*ny + 1;
    sy2 = i*ny;

    ru1 = (i-1)*nu + 1;
    ru2 = i*nu;

    Sbar(sy1:sy2,sy1:sy2) = S;
    Rbar(ru1:ru2,ru1:ru2) = R;

end

Rref = zeros(ny*H,1);

for i = 1:H

    row1 = (i-1)*ny + 1;
    row2 = i*ny;

    Rref(row1:row2) = r;
end

Xfree = Phi*x + Dbar;

Dmat = zeros(nu*H,nu*H);
UpreviousBar = zeros(nu*H,1);

for i = 1:H

    row1 = (i-1)*nu + 1;
    row2 = i*nu;

    Dmat(row1:row2,row1:row2) = eye(nu);

    if i == 1

        UpreviousBar(row1:row2) = uPrevious;

    else

        col1 = (i-2)*nu + 1;
        col2 = (i-1)*nu;

        Dmat(row1:row2,col1:col2) = -eye(nu);

    end
end

regularization = 1e-8;

G = Gamma'*Sbar*Gamma ...
    + Dmat'*Rbar*Dmat ...
    + regularization*eye(nu*H);

F = Gamma'*Sbar*(Xfree-Rref) ...
    - Dmat'*Rbar*UpreviousBar;

G = 0.5*(G+G');

U = zeros(nu*H,1);

maxRowSum = 0.0;

for i = 1:(nu*H)

    rowSum = 0.0;

    for j = 1:(nu*H)
        rowSum = rowSum + abs(G(i,j));
    end

    if rowSum > maxRowSum
        maxRowSum = rowSum;
    end
end

alpha = 1.0/max(maxRowSum,1e-9);

for iter = 1:Niter

    grad = G*U + F;

    Unew = U - alpha*grad;

    for k = 1:(nu*H)

        if Unew(k) < 0.0
            Unew(k) = 0.0;
        elseif Unew(k) > Qmax
            Unew(k) = Qmax;
        end
    end

    U = Unew;
end

q1 = U(1);
q2 = U(2);

uApplied = [q1;q2];

uPrevious = uApplied;

xPredPrevious = Ad*x + Bd*uApplied + dLearned;

plotData = zeros(14,1);

% 水位
plotData(1) = h1;
plotData(2) = h2;
plotData(3) = h3;

% 参考值
plotData(4) = r1;
plotData(5) = r2;
plotData(6) = r3;

% 控制输入
plotData(7) = q1;
plotData(8) = q2;

% Residual
plotData(9)  = residualHat(1);
plotData(10) = residualHat(2);
plotData(11) = residualHat(3);

% Prediction Error
plotData(12) = predictionError(1);
plotData(13) = predictionError(2);
plotData(14) = predictionError(3);

end


function [Ad,Bd,dd] = linearModelAffine(...
    xbar,ubar,Ts,A,C1,C2,C3,g)

epsv = 1e-6;

h1 = max(xbar(1),0.0);
h2 = max(xbar(2),0.0);
h3 = max(xbar(3),0.0);

d13 = h1-h3;
d32 = h3-h2;

absD13 = max(abs(d13),epsv);
absD32 = max(abs(d32),epsv);
h2safe = max(h2,epsv);

k13 = C1*g/sqrt(2.0*g*absD13);
k32 = C2*g/sqrt(2.0*g*absD32);
k20 = C3*g/sqrt(2.0*g*h2safe);

Ac = zeros(3,3);

Ac(1,1) = -k13/A;
Ac(1,3) =  k13/A;

Ac(2,2) = (-k32-k20)/A;
Ac(2,3) =  k32/A;

Ac(3,1) =  k13/A;
Ac(3,2) =  k32/A;
Ac(3,3) = (-k13-k32)/A;

Bc = [1.0/A  0.0;
      0.0    1.0/A;
      0.0    0.0];

% Ad = I + Ts*Ac
% Bd = Ts*Bc

Ad = eye(3) + Ts*Ac;
Bd = Ts*Bc;

fbar = nonlinearDynamics(...
    xbar,ubar,A,C1,C2,C3,g);

% dd = xbar + Ts*f(xbar,ubar) - Ad*xbar - Bd*ubar

dd = xbar + Ts*fbar - Ad*xbar - Bd*ubar;

end


function xdot = nonlinearDynamics(...
    x,u,A,C1,C2,C3,g)

h1 = max(x(1),0.0);
h2 = max(x(2),0.0);
h3 = max(x(3),0.0);

d13 = h1-h3;
d32 = h3-h2;

q13 = C1*sign(d13)*sqrt(2.0*g*abs(d13));
q32 = C2*sign(d32)*sqrt(2.0*g*abs(d32));
q20 = C3*sqrt(2.0*g*h2);

xdot = zeros(3,1);

xdot(1) = (u(1)-q13)/A;
xdot(2) = (u(2)+q32-q20)/A;
xdot(3) = (q13-q32)/A;

end

== matlab function Copy_of_control_main/Variant Subsystem/RL/ RL ==
  data: h1 input; q1 output; h2 input; h3 input; r1 input; r2 input; r3 input; q2 output
function [q1,q2] = RLcontroller(h1,h2,h3,r1,r2,r3)
%#codegen

%% Physical values
x = [h1;h2;h3];
ref = [r1;r2;r3];

%% Tracking error
e = ref-x;

%% IMPORTANT:
% Exactly the same observation used during training
obs = [
    x/60;
    e/30
];

%% Trained SAC policy
a = tankSACPolicy(obs);

%% Safety clipping
a = min(max(a,-1),1);

%% Convert normalized action [-1,1]
% to physical pump flow [0,85] ml/s

Qmax = 85;

u = (Qmax/2)*(a+1);

%% Outputs
q1 = u(1);
q2 = u(2);

end

== matlab function Copy_of_control_main/Variant Subsystem/Learning based Backstepping MIMO/MATLAB Function ==
  data: t input; q1 output; h1 input; h2 input; h3 input; r1 input; r3 input; K1 input; K3 input; Kz input; az input; q2 output; dq13 output; dq32 output; dq20 output
function [q1,q2, dq13,dq32,dq20] = Learning_based_Backstepping_MIMO( ...
    t,h1,h2,h3,r1,r3,K1,K3,Kz,az)

A = 154.0;
Sn = 0.5;
g = 981.0;
TWOG = 2*g;
epsv = 1e-6;

az1 = az(1);
az2 = az(2);
az3 = az(3);

persistent d13 d32 d20
persistent h1_old h2_old h3_old
persistent q1_old q2_old t_old
persistent initialized

if isempty(initialized)
    d13 = 0.0;
    d32 = 0.0;
    d20 = 0.0;

    h1_old = h1;
    h2_old = h2;
    h3_old = h3;

    q1_old = 0.0;
    q2_old = 0.0;
    t_old = t;

    initialized = false;
end

hdot1 = 0.0;
hdot3 = 0.0;

if initialized
    dt = t-t_old;

    if dt > epsv
        hdot1 = (h1-h1_old)/dt;
        hdot2 = (h2-h2_old)/dt;
        hdot3 = (h3-h3_old)/dt;

        h1_mid = 0.5*(h1+h1_old);
        h2_mid = 0.5*(h2+h2_old);
        h3_mid = 0.5*(h3+h3_old);

        q13_model_old = az1*Sn*sqrt(TWOG*max(h1_mid-h3_mid,0));
        q32_model_old = az3*Sn*sqrt(TWOG*max(h3_mid-h2_mid,0));
        q20_model_old = az2*Sn*sqrt(TWOG*max(h2_mid,0));

        q13_real = q1_old-A*hdot1;
        q32_real = q13_real-A*hdot3;
        q20_real = q2_old+q32_real-A*hdot2;

        target13 = q13_real-q13_model_old;
        target32 = q32_real-q32_model_old;
        target20 = q20_real-q20_model_old;

        target13 = min(max(target13,-20),20);
        target32 = min(max(target32,-20),20);
        target20 = min(max(target20,-20),20);

        gamma13 = 1.0;
        gamma32 = 1.0;
        gamma20 = 1.0;

        eta13 = 1-exp(-gamma13*dt);
        eta32 = 1-exp(-gamma32*dt);
        eta20 = 1-exp(-gamma20*dt);

        d13 = d13-eta13*(d13-target13);
        d32 = d32-eta32*(d32-target32);
        d20 = d20-eta20*(d20-target20);

        d13 = min(max(d13,-20),20);
        d32 = min(max(d32,-20),20);
        d20 = min(max(d20,-20),20);
    end
end

dq13 = d13;
dq32 = d32;
dq20 = d20;

q13_model = az1*Sn*sqrt(TWOG*max(h1-h3,0));
q32_model = az3*Sn*sqrt(TWOG*max(h3-h2,0));
q20_model = az2*Sn*sqrt(TWOG*max(h2,0));

q13 = max(q13_model+dq13,0);
q32 = max(q32_model+dq32,0);
q20 = max(q20_model+dq20,0);

e1 = h1-r1;

q1 = q13-A*K1*e1;
q1 = min(max(q1,0),85);

e3 = h3-r3;

q32_des = q13+A*K3*e3;

z = q32-q32_des;

dh13 = max(h1-h3,epsv);
dh32 = max(h3-h2,epsv);

k13 = (az1*Sn*TWOG)/(2*sqrt(TWOG*dh13));
k32 = (az3*Sn*TWOG)/(2*sqrt(TWOG*dh32));

k32 = max(k32,1e-3);

q13_dot = k13*(hdot1-hdot3);

q32_des_dot = q13_dot+A*K3*hdot3;

q2 = q13-2*q32+q20 ...
    -(A/k32)*q32_des_dot ...
    +(A/k32)*Kz*z;

q2 = min(max(q2,0),85);

h1_old = h1;
h2_old = h2;
h3_old = h3;

q1_old = q1;
q2_old = q2;
t_old = t;

initialized = true;

end

== matlab function Copy_of_control_main/Variant Subsystem/Learning based IO Linearization MIMO/MATLAB Function ==
  data: t input; q1 output; h1 input; h2 input; h3 input; r1 input; r3 input; Kp1 input; Kp3 input; Kd3 input; az input; q2 output; dq13 output; dq32 output; dq20 output
function [q1,q2,dq13,dq32,dq20] = ...
    Learning_based_IO_MIMO( ...
    t,h1,h2,h3,r1,r3,Kp1,Kp3,Kd3,az)

% =========================================================
% Three-tank learning-based input-output linearization
%
% Inputs:
%   t              simulation time from Clock block
%   h1,h2,h3       measured liquid levels
%   r1,r3          references
%   Kp1            proportional gain for h1
%   Kp3,Kd3        PD gains for h3
%   az             discharge coefficients [az1 az2 az3]
%
% Outputs:
%   q1,q2          pump inputs
%   dq13,dq32,dq20 learned flow residuals
% =========================================================

%% Physical parameters
% Use the same numerical values as in your original program
A     = 154;       % Tank cross-sectional area
Sn    = 0.5;       % Outlet cross-sectional area
TWOG  = 1962;      % 2*g, depending on your unit system

az1 = az(1);
az2 = az(2);
az3 = az(3);

%% Residual-learning parameters
% Larger gamma means faster adaptation but more sensitivity to noise
gamma13 = 0.5;
gamma32 = 0.5;
gamma20 = 0.5;

%% Persistent variables
persistent d13 d32 d20
persistent h1_old h2_old h3_old
persistent q1_old q2_old
persistent e3_old
persistent t_old
persistent initialized

%% Initialization
if isempty(initialized)

    % Initial residual estimates
    d13 = 0.0;
    d32 = 0.0;
    d20 = 0.0;

    % Initial measured levels
    h1_old = h1;
    h2_old = h2;
    h3_old = h3;

    % Initial pump inputs
    q1_old = 0.0;
    q2_old = 0.0;

    % Initialize derivative calculation
    e3_old = r3-h3;
    t_old  = t;

    initialized = true;
end

%% Actual elapsed time
dt = t-t_old;

% Prevent division by zero or negative solver time steps
if dt < 1e-8
    dt = 0.0;
end

%% ========================================================
% 1. Online residual estimation
% =========================================================

if dt > 0

    % Estimate liquid-level derivatives
    hdot1 = (h1-h1_old)/dt;
    hdot2 = (h2-h2_old)/dt;
    hdot3 = (h3-h3_old)/dt;

    % Midpoint levels approximate the average state over
    % the previous sampling interval
    h1_mid = 0.5*(h1+h1_old);
    h2_mid = 0.5*(h2+h2_old);
    h3_mid = 0.5*(h3+h3_old);

    % Nominal flow models over the previous interval
    q13_model_old = az1*Sn*sqrt( ...
        TWOG*max(h1_mid-h3_mid,0));

    q32_model_old = az3*Sn*sqrt( ...
        TWOG*max(h3_mid-h2_mid,0));

    q20_model_old = az2*Sn*sqrt( ...
        TWOG*max(h2_mid,0));

    % -----------------------------------------------------
    % Reconstruct actual flows from mass conservation
    %
    % A*hdot1 = q1-q13
    % A*hdot3 = q13-q32
    % A*hdot2 = q2+q32-q20
    % -----------------------------------------------------

    q13_real = q1_old-A*hdot1;

    q32_real = q13_real-A*hdot3;

    q20_real = q2_old+q32_real-A*hdot2;

    % Residual targets
    target13 = q13_real-q13_model_old;
    target32 = q32_real-q32_model_old;
    target20 = q20_real-q20_model_old;

    % Continuous-rate-compatible learning factors
    eta13 = 1-exp(-gamma13*dt);
    eta32 = 1-exp(-gamma32*dt);
    eta20 = 1-exp(-gamma20*dt);

    % Exponentially smoothed online residual estimates
    d13 = d13+eta13*(target13-d13);
    d32 = d32+eta32*(target32-d32);
    d20 = d20+eta20*(target20-d20);
end

%% ========================================================
% 2. Current nominal flow models
% =========================================================

dh13 = max(h1-h3,0);
dh32 = max(h3-h2,0);
dh20 = max(h2,0);

q13_model = az1*Sn*sqrt(TWOG*dh13);
q32_model = az3*Sn*sqrt(TWOG*dh32);
q20_model = az2*Sn*sqrt(TWOG*dh20);

%% ========================================================
% 3. Residual-compensated flow models
% =========================================================

q13 = q13_model+d13;
q32 = q32_model+d32;
q20 = q20_model+d20;

% Optional physical protection against negative flow estimates
q13 = max(q13,0);
q32 = max(q32,0);
q20 = max(q20,0);

%% ========================================================
% 4. Corrected q1 input-output linearization
% =========================================================

e1 = r1-h1;

% Since A*hdot1 = q1-q13, choose:
%
% hdot1 = Kp1*(r1-h1)
%
% Therefore:
% q1 = q13 + A*Kp1*e1

q1 = q13+A*Kp1*e1;

% Pump saturation
q1 = min(max(q1,0),85);

%% ========================================================
% 5. Nonlinear coefficients for the h3 channel
% =========================================================

% A small lower bound prevents numerical division by zero
epsilon = 1e-6;

den13 = sqrt(TWOG*dh13+epsilon);
den32 = sqrt(TWOG*dh32+epsilon);

% k1 = alpha13/alpha32
k1 = az1*den32/(az3*den13);

% k2 = alpha32 = derivative of q32 with respect to h3-h2
k2 = TWOG*az3*Sn/(2*den32);

%% ========================================================
% 6. PD virtual input for h3
% =========================================================

e3 = r3-h3;

if dt > 0
    e3_dot = (e3-e3_old)/dt;
else
    e3_dot = 0.0;
end

pd = Kp3*e3+Kd3*e3_dot;

%% ========================================================
% 7. Input-output linearization for q2
% =========================================================

q2 = -k1*(q1-2*q13+q32) ...
     +(q13-2*q32+q20) ...
     +(A*A/k2)*pd;

% Pump saturation
q2 = min(max(q2,0),85);

%% ========================================================
% 8. Save values for the next sampling instant
% =========================================================

h1_old = h1;
h2_old = h2;
h3_old = h3;

q1_old = q1;
q2_old = q2;

e3_old = e3;
t_old  = t;

%% Residual outputs
dq13 = d13;
dq32 = d32;
dq20 = d20;

end

== matlab function Copy_of_control_main/MATLAB Function1 ==
  data: dac1 input; packet output; dac2 input
function packet = buildPacket(dac1, dac2)

% dac1 = uint8(0);
% dac2 = uint8(0);

packet = uint8(zeros(5,1));
packet(1) = hex2dec('BB');
packet(2) = hex2dec('02');
packet(3) = dac1;
packet(4) = dac2;

checksum = uint8(0);
for i = 1:4
    checksum = bitxor(checksum, packet(i));
end
packet(5) = checksum;

== matlab function Copy_of_control_main/MATLAB Function ==
  data: packet input; adc1 output; adc2 output; adc3 output; valid output
function [adc1, adc2, adc3, valid] = parsePacket(packet)

checksum = uint8(0);
for i = 1:6
    checksum = bitxor(checksum, uint8(packet(i)));
end

if checksum == uint8(packet(7))
    adc1 = double(bitshift(uint16(packet(1)), 8) + uint16(packet(2))) * (3.3 / 4095);
    adc2 = double(bitshift(uint16(packet(3)), 8) + uint16(packet(4))) * (3.3 / 4095);
    adc3 = double(bitshift(uint16(packet(5)), 8) + uint16(packet(6))) * (3.3 / 4095);
    valid = true;
else
    adc1 = 0;
    adc2 = 0;
    adc3 = 0;
    valid = false;
end

end

== matlab function Copy_of_control_main/ADC_to_Height ==
  data: adc1 input; h1 output; adc2 input; adc3 input; c input; h2 output; h3 output
function [h1,h2,h3] = fcn(adc1,adc2,adc3,c)

h1 = c(1,1)*adc1^3 + c(1,2)*adc1^2 + c(1,3)*adc1 + c(1,4);
h2 = c(2,1)*adc3^3 + c(2,2)*adc3^2 + c(2,3)*adc3 + c(2,4);
h3 = c(3,1)*adc2^3 + c(3,2)*adc2^2 + c(3,3)*adc2 + c(3,4);

end

== matlab function Copy_of_control_main/Q_to_DAC ==
  data: q1 input; dac1 output; q2 input; Q input; dac2 output
function [dac1,dac2] = fcn(q1,q2,Q)

dac_table = [255 223 191 159 128 96 64 32 0];

q1 = min(max(q1, Q(1,1)), Q(1,end));
q2 = min(max(q2, Q(2,1)), Q(2,end));

dac1 = interp1(Q(1,:), dac_table, q1, 'linear');
dac2 = interp1(Q(2,:), dac_table, q2, 'linear');

dac1 = min(max(dac1,0),255);
dac2 = min(max(dac2,0),255);

end

== matlab function Copy_of_control_main/Variant Subsystem/PI MIMO/MATLAB Function ==
  data: h1 input; h3 input; r1 input; r3 input; Kp1 input; Ki1 input; q1 output; Kp3 input; Ki3 input; q2 output
function [q1, q2] = PI_MIMO_T1T3(h1, h3, r1, r3, Kp1, Ki1, Kp3, Ki3)
%#codegen

persistent q1_old e1_old
persistent q2_old e3_old

if isempty(q1_old)
    q1_old = 0;
    e1_old = 0;
    q2_old = 0;
    e3_old = 0;
end

Ts = 0.01;

% PI loop 1: h1 -> q1
e1 = r1 - h1;
k1 = Ki1 * Ts / 2;
zk10 = Kp1 + k1;
zk11 = k1 - Kp1;

q1_new = q1_old + zk10 * e1 + zk11 * e1_old;
q1_new = min(max(q1_new, 0), 85);

% PI loop 2: h3 -> q2
e3 = r3 - h3;
k3 = Ki3 * Ts / 2;
zk30 = Kp3 + k3;
zk31 = k3 - Kp3;

q2_new = q2_old + zk30 * e3 + zk31 * e3_old;
q2_new = min(max(q2_new, 0), 85);

q1 = q1_new;
q2 = q2_new;

q1_old = q1_new;
e1_old = e1;

q2_old = q2_new;
e3_old = e3;

end

== matlab function Copy_of_control_main/Variant Subsystem/PI SISO/MATLAB Function ==
  data: h2 input; q1 output; r2 input; Kp input; Ki input; q2 output
function [q1,q2] = PI_SISO(h2,r2,Kp,Ki)

persistent u_old e_old

if isempty(u_old)
    u_old = 0;
    e_old = 0;
end

% ESP32 sample time: 100 Hz = 0.01 s
Ts = 0.01;

e = r2 - h2;

k = Ki * Ts / 2;
zk0 = Kp + k;
zk1 = k - Kp;

u = u_old + zk0 * e + zk1 * e_old;

u = min(max(u, 0), 85);

q1 = 0;
q2 = u;

u_old = u;
e_old = e;

end

== matlab function Copy_of_control_main/Variant Subsystem/IO Linearization SISO/MATLAB Function ==
  data: h2 input; q1 output; r2 input; Kp input; az input; q2 output
function [q1,q2] = IO_SISO(h2,r2,Kp,az)

A  = 154;
Sn = 0.5;
g  = 981;

Ofc2 = az(2);

e = r2 - h2;

% IO linearization
q1 = 0;
q2 = A*Kp*e + Ofc2*Sn*sqrt(2*g*max(h2,0));

q2 = min(max(q2,0),85);

end
